simulink model "controllo_LQ_inseguimento"  (R2021a)
settings: Solver=VariableStepAuto  StartTime=0.0  StopTime=tsim  RelTol=1e-3
values from neighbouring files (symbols this model uses):
  Arc = 0    [main.m]
  b = 20    [main.m]
  Brc = 0    [main.m]
  c = 718    [main.m]
  F_fb = F_aug (:,1:nx)    [main.m]
  F_ff = F_aug (:, nx+1:end)    [main.m]
  f_w = 0    [main.m]
  g = 9.81    [main.m]
  k = 2.5    [main.m]
  m = 500    [main.m]
  p_a = 1.184    [main.m]
  Tc = 0.01    [main.m]
  theta_a = 298    [main.m]
  u_eq = k*(theta - theta_a)    (= 199.411134904)    [main.m]
  V = 2000    [main.m]
  x_0 = [550;0;150]    [main.m]
  x_eq = [600;0;theta]    [main.m]
undefined symbols (not defined in the file or in its folder): Cd, nr
settings Model: Creator=Randy  LastModifiedBy=Randy

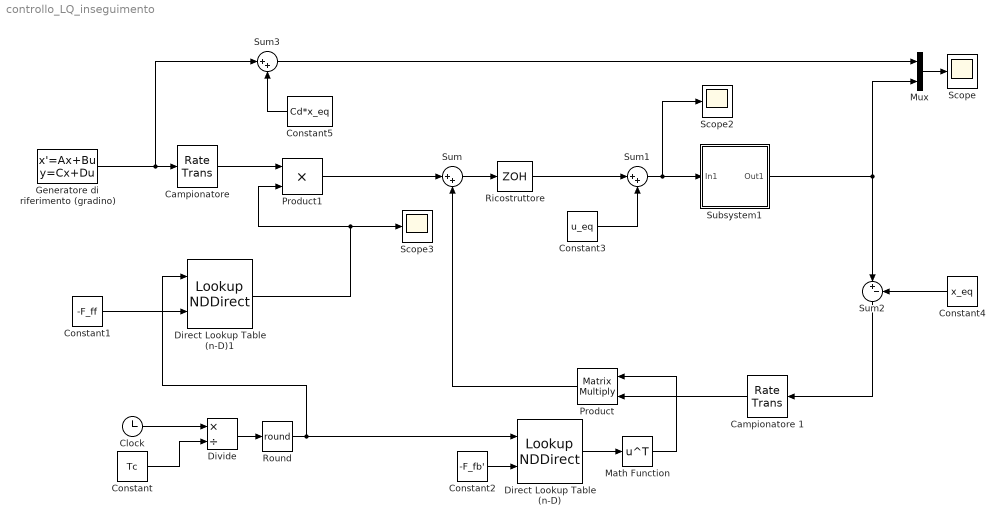
== system controllo_LQ_inseguimento ==
  Campionatore : RateTransition  OutPortSampleTime=Tc
  Campionatore 1 : RateTransition  OutPortSampleTime=Tc
  Clock : Clock
  Constant : Constant  Value=Tc
  Constant1 : Constant  Value=-F_ff  VectorParams1D=off
  Constant2 : Constant  Value=-F_fb'  VectorParams1D=off
  Constant3 : Constant  Value=u_eq
  Constant4 : Constant  Value=x_eq
  Constant5 : Constant  Value=Cd*x_eq
  Direct Lookup Table (n-D) : LookupNDDirect  InputsSelectThisObjectFromTable=Vector  TableIsInput=on  Table=-F_fb'
  Direct Lookup Table (n-D)1 : LookupNDDirect  NumberOfTableDimensions=1  TableIsInput=on  Table=-F_ff'
  Divide : Product  Inputs=*/
  Generatore di riferimento (gradino) : StateSpace  A=Arc  B=Brc  C=eye(nr)  D=0  InitialCondition=0  ParameterTunability=Unconstrained
  Math Function : Math  Operator=transpose  SaturateOnIntegerOverflow=on
  Mux : Mux  Inputs=2
  Product : Product  Multiplication=Matrix(*)
  Product1 : Product
  Ricostruttore : ZeroOrderHold  SampleTime=-1
  Round : Rounding  Operator=round
  Scope : Scope
  Scope2 : Scope
  Scope3 : Scope
  Subsystem1 : Subsystem
  Sum : Sum  Inputs=|++
  Sum1 : Sum  Inputs=|++
  Sum2 : Sum  Inputs=|+-
  Sum3 : Sum  Inputs=|++
  wires:
  Subsystem1/1(Out1) -> Mux/2, Sum2/1
  Direct Lookup Table (n-D)/1 -> Math Function/1
  Math Function/1 -> Product/1
  Campionatore 1/1 -> Product/2
  Divide/1 -> Round/1
  Round/1 -> Direct Lookup Table (n-D)1/1, Direct Lookup Table (n-D)/1
  Clock/1 -> Divide/1
  Constant/1 -> Divide/2
  Generatore di riferimento (gradino)/1 -> Sum3/1, Campionatore/1
  Constant1/1 -> Direct Lookup Table (n-D)1/2
  Constant2/1 -> Direct Lookup Table (n-D)/2
  Sum/1 -> Ricostruttore/1
  Sum1/1 -> Scope2/1, Subsystem1/1(In1)
  Constant3/1 -> Sum1/2
  Sum2/1 -> Campionatore 1/1
  Constant4/1 -> Sum2/2
  Direct Lookup Table (n-D)1/1 -> Product1/2, Scope3/1
  Product1/1 -> Sum/1
  Campionatore/1 -> Product1/1
  Ricostruttore/1 -> Sum1/1
  Product/1 -> Sum/2
  Constant5/1 -> Sum3/2
  Sum3/1 -> Mux/1
  Mux/1 -> Scope/1

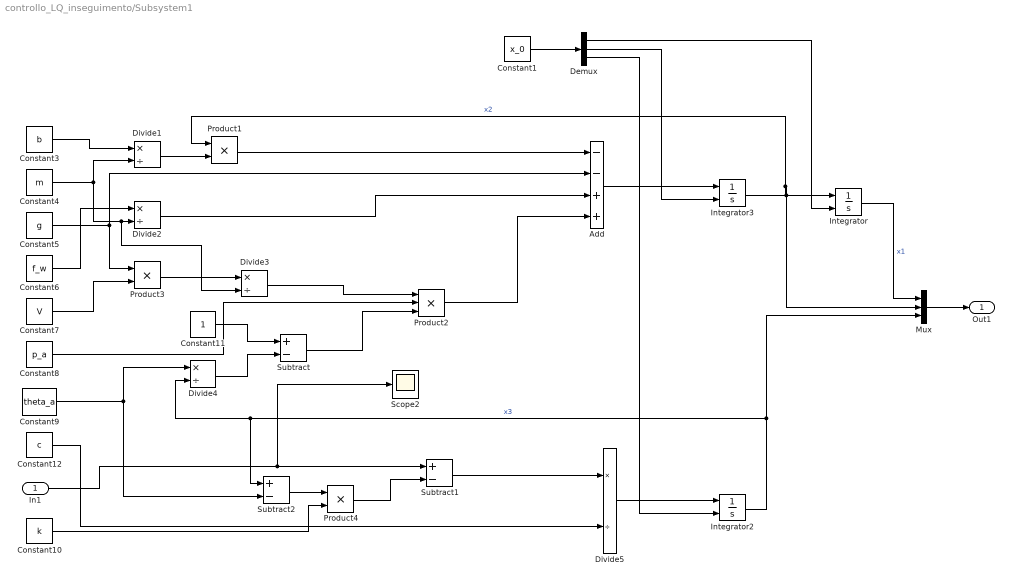
== system controllo_LQ_inseguimento/Subsystem1 ==
  In1 : Inport
  Add : Sum  Inputs=--++
  Constant1 : Constant  Value=x_0
  Constant10 : Constant  Value=k
  Constant11 : Constant
  Constant12 : Constant  Value=c
  Constant3 : Constant  Value=b
  Constant4 : Constant  Value=m
  Constant5 : Constant  Value=g
  Constant6 : Constant  Value=f_w
  Constant7 : Constant  Value=V
  Constant8 : Constant  Value=p_a
  Constant9 : Constant  Value=theta_a
  Demux : Demux  Outputs=3
  Divide{1..5} (5 alike) : Product  Inputs=*/
  Integrator : Integrator  InitialConditionSource=external  InitialCondition=680
  Integrator2 : Integrator  InitialConditionSource=external  InitialCondition=400
  Integrator3 : Integrator  InitialConditionSource=external
  Mux : Mux  Inputs=3
  Product1 : Product
  Product2 : Product  Inputs=3
  Product3 : Product
  Product4 : Product
  Scope2 : Scope
  Subtract : Sum  Inputs=+-
  Subtract1 : Sum  Inputs=+-
  Subtract2 : Sum  Inputs=+-
  Out1 : Outport
  wires:
  Subtract/1 -> Product2/3
  In1/1 -> Scope2/1, Subtract1/1
  Constant9/1 -> Subtract2/2, Divide4/1
  Constant5/1 -> Product3/1, Add/2
  Divide4/1 -> Subtract/2
  Constant10/1 -> Product4/2
  Constant7/1 -> Product3/2
  Product2/1 -> Add/4
  Subtract2/1 -> Product4/1
  Divide1/1 -> Product1/2
  Constant3/1 -> Divide1/1
  Product4/1 -> Subtract1/2
  Constant11/1 -> Subtract/1
  Integrator3/1 -> Mux/2, Integrator/1, Product1/1  "x2"
  Divide2/1 -> Add/3
  Integrator/1 -> Mux/1  "x1"
  Constant4/1 -> Divide3/2, Divide2/2, Divide1/2
  Product3/1 -> Divide3/1
  Product1/1 -> Add/1
  Divide3/1 -> Product2/1
  Mux/1 -> Out1/1
  Add/1 -> Integrator3/1
  Constant8/1 -> Product2/2
  Divide5/1 -> Integrator2/1
  Constant12/1 -> Divide5/2
  Constant6/1 -> Divide2/1
  Subtract1/1 -> Divide5/1
  Integrator2/1 -> Mux/3, Subtract2/1, Divide4/2  "x3"
  Constant1/1 -> Demux/1
  Demux/1 -> Integrator/2
  Demux/2 -> Integrator3/2
  Demux/3 -> Integrator2/2
